simulink model "Circuito_RLC"  (R2020a)
settings: Solver=VariableStepAuto  StartTime=0.0  StopTime=10.0  RelTol=1e-3
values from neighbouring files (symbols this model uses):
  c = 1    [CircuitoRLC.m]
  l = 1    [CircuitoRLC.m]
  r = 1    [CircuitoRLC.m]
  v = 10    [CircuitoRLC.m]
settings Model: Creator=gabri  LastModifiedBy=gabri

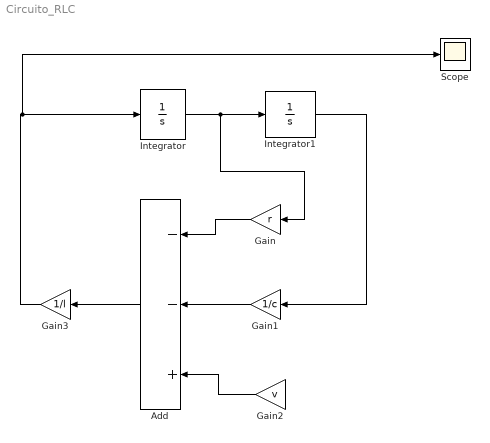
== system Circuito_RLC ==
  Add : Sum  Inputs=--+
  Gain : Gain  Gain=r
  Gain1 : Gain  Gain=1/c
  Gain2 : Gain  Gain=v
  Gain3 : Gain  Gain=1/l
  Integrator : Integrator
  Integrator1 : Integrator  InitialCondition=10
  Scope : Scope
  wires:
  Integrator/1 -> Gain/1, Integrator1/1
  Gain3/1 -> Scope/1, Integrator/1
  Integrator1/1 -> Gain1/1
  Gain/1 -> Add/1
  Gain1/1 -> Add/2
  Gain2/1 -> Add/3
  Add/1 -> Gain3/1
